simulink model "set_speed"  (R2021b)
settings: Solver=FixedStepDiscrete  StartTime=0.0  StopTime=inf  FixedStep=0.05  RelTol=1e-3
InitFcn:
  | ONE_FLOAT=1;
  | KVDI_ACCSetSpdIntial_kph=30;
  | KVDI_ACCLongPressTime_ms=3000;
  | KVDI_LongPressConTime_ms=800;
  | KVDI_ACCSpdLargeChange_kph=5;
  | ZERO_FLOAT=0;
  | FALSE=0;
  | TRUE=1;
  | ENUM_ACCSTATE_OFF=0;
  | ENUM_ACCSTATE_DISABLED=0;
  | ENUM_ACCSTATE_STANDBY=1;
  | KVDI_ACCMaxActSpeed_kph=150;
  | ONE_INT=1;
  | ZERO_INT=0;
  | C_TICK_TIME_S=0.05;
libraries: realtime_pacer_lib x1, simulink x1
settings Model: Creator=ZHEN-YU  LastModifiedBy=ZHEN-YU

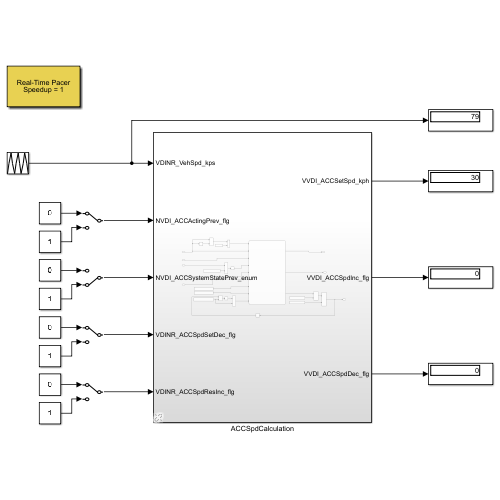
[thumbnail: Simulink's stored preview of the top-level diagram]
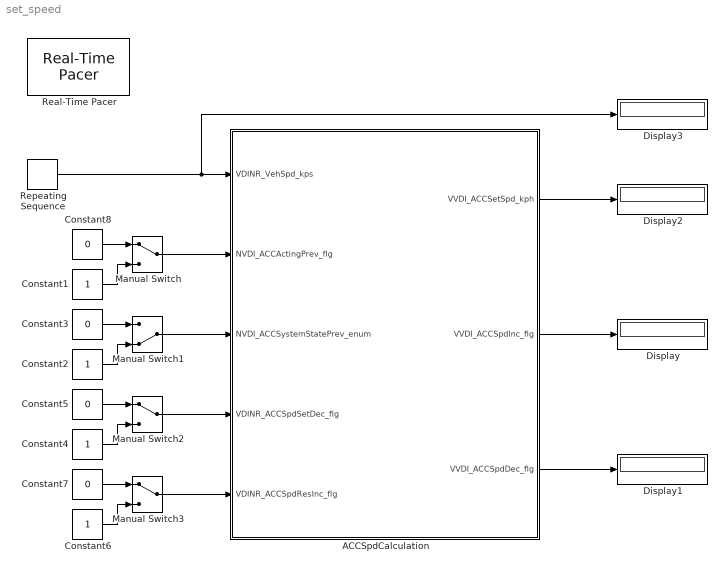
== system set_speed ==
  ACCSpdCalculation : Subsystem  AncestorBlock=vdi_v5/IFO/VDI/ACC/ACCSpdCalculation
  Constant{1..2,4,6} (4 alike) : Constant  OutDataTypeStr=boolean
  Constant{3,5,7..8} (4 alike) : Constant  Value=0  OutDataTypeStr=boolean
  Display{,1..3} (4 alike) : Display
  Manual Switch : ManualSwitch
  Manual Switch1 : ManualSwitch  CurrentSetting=0
  Manual Switch2 : ManualSwitch
  Manual Switch3 : ManualSwitch
  Real-Time Pacer : realtime_pacer_lib/Real-Time Pacer  simTimePerRealTime=1
  Repeating Sequence : simulink/Sources/Repeating Sequence  rep_seq_t=[0 10 20 30 40]  rep_seq_y=[0 50 100 50 0]
  wires:
  Repeating Sequence/1 -> Display3/1, ACCSpdCalculation/1(VDINR_VehSpd_kps)
  ACCSpdCalculation/2(VVDI_ACCSpdInc_flg) -> Display/1
  ACCSpdCalculation/3(VVDI_ACCSpdDec_flg) -> Display1/1
  ACCSpdCalculation/1(VVDI_ACCSetSpd_kph) -> Display2/1
  Constant8/1 -> Manual Switch/1
  Constant1/1 -> Manual Switch/2
  Manual Switch/1 -> ACCSpdCalculation/2(NVDI_ACCActingPrev_flg)
  Constant2/1 -> Manual Switch1/2
  Constant3/1 -> Manual Switch1/1
  Manual Switch1/1 -> ACCSpdCalculation/3(NVDI_ACCSystemStatePrev_enum)
  Constant5/1 -> Manual Switch2/1
  Constant4/1 -> Manual Switch2/2
  Manual Switch2/1 -> ACCSpdCalculation/4(VDINR_ACCSpdSetDec_flg)
  Manual Switch3/1 -> ACCSpdCalculation/5(VDINR_ACCSpdResInc_flg)
  Constant6/1 -> Manual Switch3/2
  Constant7/1 -> Manual Switch3/1

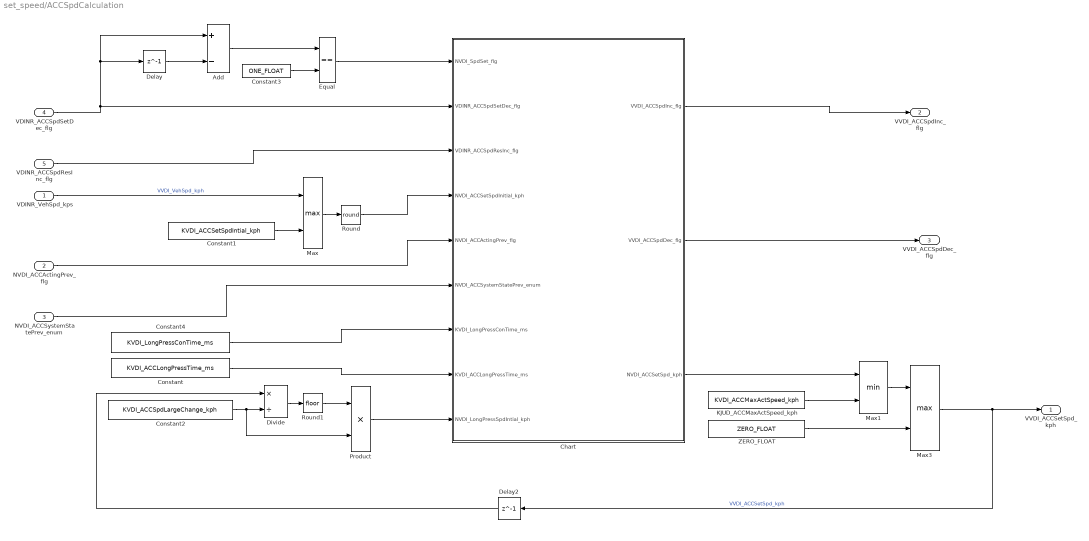
== system set_speed/ACCSpdCalculation ==
  VDINR_VehSpd_kps : Inport
  NVDI_ACCActingPrev_flg : Inport  Port=2
  NVDI_ACCSystemStatePrev_enum : Inport  Port=3
  VDINR_ACCSpdSetDec_flg : Inport  Port=4
  VDINR_ACCSpdResInc_flg : Inport  Port=5
  Add : Sum  Inputs=+-
  Chart : Stateflow chart  TreatAsAtomicUnit=on
      settings: PortSchema="{\"entries\":[{\"content\":{\"sides\":[{\"content\":{\"connectorIds\":[\"In1\",\"In2\",\"In3\",\"In4\",\"In5\",\"In6\",\"In9\",\"In7\",\"In8\"]},\"type\":\"ConnectorPlacement.EquallySpacedRectSide\",\"uuid\":\"b1b09059-7c6b-4f2a-a509-9d89abb69bff\"},{\"content\":{\"connectorIds\":[\"Out2\",\"Out3\",\"Out1\"],\"side\":\"RIGHT\"},\"type\":\"ConnectorPlacement.EquallySpacedRectSide\",\"uuid\":\"426eb2b7-8f84-437e-9ce1-b8172d5a5373\"},{\"content\":{\"connectorIds\":[],\"side\":\"TOP\"},\"type\":\"ConnectorPlacement.EquallySpacedRectSide\",\"uuid\":\"808310a0-6f78-4728-b2e8-69880cb1a9d0\"}]},\"type\":\"ConnectorPlacement.EquallySpacedConnector\",\"uuid\":\"50fcbb31-1c9a-4815-926e-b0772552613f\"}],\"packageUris\":[\"http://schema.mathworks.com/mf0/Connector/R2020b\"],\"version\":\"1.0\"}"
  Constant : Constant  Value=KVDI_ACCLongPressTime_ms
  Constant1 : Constant  Value=KVDI_ACCSetSpdIntial_kph
  Constant2 : Constant  Value=KVDI_ACCSpdLargeChange_kph
  Constant3 : Constant  Value=ONE_FLOAT
  Constant4 : Constant  Value=KVDI_LongPressConTime_ms
  Delay : Delay  DelayLength=1
  Delay2 : Delay  DelayLength=1
  Divide : Product  Inputs=*/
  Equal : RelationalOperator  Operator===  OutDataTypeStr=boolean  RndMeth=Simplest
  KJUD_ACCMaxActSpeed_kph : Constant  Value=KVDI_ACCMaxActSpeed_kph
  Max : MinMax  Function=max  Inputs=2
  Max1 : MinMax  Inputs=2
  Max3 : MinMax  Function=max  Inputs=2
  Product : Product
  Round : Rounding  Operator=round
  Round1 : Rounding
  ZERO_FLOAT : Constant  Value=ZERO_FLOAT
  VVDI_ACCSetSpd_kph : Outport
  VVDI_ACCSpdInc_flg : Outport  Port=2
  VVDI_ACCSpdDec_flg : Outport  Port=3
  wires:
  Constant/1 -> Chart/7(KVDI_ACCLongPressTime_ms)
  VDINR_ACCSpdResInc_flg/1 -> Chart/3(VDINR_ACCSpdResInc_flg)
  Max3/1 -> Delay2/1, VVDI_ACCSetSpd_kph/1  "VVDI_ACCSetSpd_kph"
  NVDI_ACCActingPrev_flg/1 -> Chart/5(NVDI_ACCActingPrev_flg)
  NVDI_ACCSystemStatePrev_enum/1 -> Chart/6(NVDI_ACCSystemStatePrev_enum)
  Max/1 -> Round/1
  Constant1/1 -> Max/2
  VDINR_VehSpd_kps/1 -> Max/1  "VVDI_VehSpd_kph"
  Round/1 -> Chart/4(NVDI_ACCSetSpdInitial_kph)
  Delay2/1 -> Divide/1
  Constant2/1 -> Product/2, Divide/2
  Round1/1 -> Product/1
  Divide/1 -> Round1/1
  Product/1 -> Chart/8(NVDI_LongPressSpdIntial_kph)
  Chart/1(NVDI_ACCSetSpd_kph) -> Max1/1
  ZERO_FLOAT/1 -> Max3/2
  Equal/1 -> Chart/1(NVDI_SpdSet_flg)
  Add/1 -> Equal/1
  Delay/1 -> Add/2
  Constant3/1 -> Equal/2
  VDINR_ACCSpdSetDec_flg/1 -> Add/1, Delay/1, Chart/2(VDINR_ACCSpdSetDec_flg)
  KJUD_ACCMaxActSpeed_kph/1 -> Max1/2
  Max1/1 -> Max3/1
  Chart/3(VVDI_ACCSpdDec_flg) -> VVDI_ACCSpdDec_flg/1
  Chart/2(VVDI_ACCSpdInc_flg) -> VVDI_ACCSpdInc_flg/1
  Constant4/1 -> Chart/9(KVDI_LongPressConTime_ms)

== stateflow chart set_speed/ACCSpdCalculation/Chart ==
  state INITIALIZATION
    en:
    NVDI_ACCSetSpd_kph = ZERO_INT;
    NVDI_ACCResSpd_kph=ZERO_INT;
    VVDI_ACCSpdDec_flg=FALSE;
    VVDI_ACCSpdInc_flg=FALSE;
  state STANDBY
    en:
    VVDI_ACCSpdDec_flg=FALSE;
    VVDI_ACCSpdInc_flg=FALSE;
    state Initial
      du:
      NVDI_ACCSetSpd_kph=NVDI_ACCSetSpdInitial_kph
    state Resume
      en:
      NVDI_ACCSetSpd_kph=NVDI_ACCResSpd_kph
    state Setting
      en:
      NVDI_ACCSetSpd_kph=NVDI_ACCSetSpdInitial_kph
    (default) -> Initial
    Initial -> Resume [order 2] : [VDINR_ACCSpdResInc_flg==TRUE...
        | &&NVDI_ACCResSpd_kph~=ZERO_INT]
    Resume -> Setting : [NVDI_SpdSet_flg==TRUE]
    Setting -> Resume : [VDINR_ACCSpdResInc_flg==TRUE...
        | &&NVDI_ACCResSpd_kph~=ZERO_INT]
    Initial -> Setting [order 1] : [NVDI_SpdSet_flg==TRUE]
  state SPEED_MODIF
    state Inc_Speed
      du:
      NVDI_ACCResSpd_kph=NVDI_ACCSetSpd_kph;
      VVDI_ACCSpdInc_flg=TRUE;
      state Small_Inc
        en:
        NVDI_ACCSetSpd_kph=NVDI_ACCSetSpd_kph+ONE_INT;
        NVDI_ACCIncTimer_ms=ZERO_INT;
        du:
        NVDI_ACCIncTimer_ms=NVDI_ACCIncTimer_ms+(C_TICK_TIME_S*1000);
      state Large_Inc_Frist
        en:
        NVDI_ACCSetSpd_kph=NVDI_LongPressSpdIntial_kph+KVDI_ACCSpdLargeChange_kph
      state MAINTAIN
        en:
        NVDI_ACCIncTimer_ms=ZERO_INT;
        du:
        NVDI_ACCIncTimer_ms=NVDI_ACCIncTimer_ms+(C_TICK_TIME_S*1000);
      state Large_Inc
        en:
        NVDI_ACCSetSpd_kph=NVDI_ACCSetSpd_kph+KVDI_ACCSpdLargeChange_kph
      (default) -> Small_Inc
      Small_Inc -> Large_Inc_Frist : [NVDI_ACCIncTimer_ms>KVDI_ACCLongPressTime_ms]
      Large_Inc_Frist -> SPEED_MODIF.Inc_Speed.MAINTAIN
      SPEED_MODIF.Inc_Speed.MAINTAIN -> Large_Inc : [NVDI_ACCIncTimer_ms>KVDI_LongPressConTime_ms]
      Large_Inc -> SPEED_MODIF.Inc_Speed.MAINTAIN
    state Dec_Speed
      du:
      NVDI_ACCResSpd_kph=NVDI_ACCSetSpd_kph;
      VVDI_ACCSpdDec_flg=TRUE;
      state Small_Dec
        en:
        NVDI_ACCSetSpd_kph=NVDI_ACCSetSpd_kph-ONE_INT;
        NVDI_ACCDecTimer_ms=ZERO_INT;
        du:
        NVDI_ACCDecTimer_ms=NVDI_ACCDecTimer_ms+(C_TICK_TIME_S*1000);
      state Large_Dec_Frist
        en:
        NVDI_ACCSetSpd_kph=NVDI_LongPressSpdIntial_kph
      state MAINTAIN
        en:
        NVDI_ACCDecTimer_ms=ZERO_INT;
        du:
        NVDI_ACCDecTimer_ms=NVDI_ACCDecTimer_ms+(C_TICK_TIME_S*1000);
      state Large_Dec
        en:
        NVDI_ACCSetSpd_kph=NVDI_ACCSetSpd_kph-KVDI_ACCSpdLargeChange_kph
      (default) -> Small_Dec
      Small_Dec -> Large_Dec_Frist : [NVDI_ACCDecTimer_ms>KVDI_ACCLongPressTime_ms]
      Large_Dec_Frist -> SPEED_MODIF.Dec_Speed.MAINTAIN
      Large_Dec -> SPEED_MODIF.Dec_Speed.MAINTAIN
      SPEED_MODIF.Dec_Speed.MAINTAIN -> Large_Dec : [NVDI_ACCDecTimer_ms>KVDI_LongPressConTime_ms]
    state HOLD
      en:
      NVDI_ACCSetSpd_kph=NVDI_ACCSetSpd_kph
      NVDI_ACCResSpd_kph=NVDI_ACCSetSpd_kph;
      VVDI_ACCSpdDec_flg=FALSE;
      VVDI_ACCSpdInc_flg=FALSE;
    (default) -> HOLD
    HOLD -> Dec_Speed [order 1] : [VDINR_ACCSpdSetDec_flg==TRUE]
    HOLD -> Inc_Speed [order 2] : [VDINR_ACCSpdResInc_flg==TRUE]
    Dec_Speed -> HOLD : [VDINR_ACCSpdSetDec_flg==FALSE]
    Inc_Speed -> HOLD : [VDINR_ACCSpdResInc_flg==FALSE]
  (default) -> INITIALIZATION
  INITIALIZATION -> STANDBY : [NVDI_ACCSystemStatePrev_enum == ENUM_ACCSTATE_STANDBY]
  STANDBY -> SPEED_MODIF [order 2] : [NVDI_ACCActingPrev_flg==TRUE]
  STANDBY -> INITIALIZATION [order 1] : [NVDI_ACCSystemStatePrev_enum == ENUM_ACCSTATE_OFF...
      | || NVDI_ACCSystemStatePrev_enum == ENUM_ACCSTATE_DISABLED]
  SPEED_MODIF -> STANDBY [order 2] : [NVDI_ACCActingPrev_flg==FALSE]
  SPEED_MODIF -> INITIALIZATION [order 1] : [NVDI_ACCSystemStatePrev_enum == ENUM_ACCSTATE_OFF...
      | || NVDI_ACCSystemStatePrev_enum == ENUM_ACCSTATE_DISABLED]
  data: NVDI_SpdSet_flg input; VDINR_ACCSpdSetDec_flg input; VDINR_ACCSpdResInc_flg input; NVDI_ACCSetSpdInitial_kph input; NVDI_ACCActingPrev_flg input; NVDI_ACCSystemStatePrev_enum input; NVDI_ACCSetSpd_kph output; KVDI_ACCLongPressTime_ms input; NVDI_LongPressSpdIntial_kph input; TRUE parameter boolean; ZERO_INT parameter; ONE_INT parameter; FALSE parameter boolean; ENUM_ACCSTATE_STANDBY parameter; ENUM_ACCSTATE_OFF parameter; ENUM_ACCSTATE_DISABLED parameter; C_TICK_TIME_S parameter; NVDI_ACCIncTimer_ms local; NVDI_ACCDecTimer_ms local; KVDI_ACCSpdLargeChange_kph parameter; NVDI_ACCResSpd_kph local; VVDI_ACCSpdInc_flg output; VVDI_ACCSpdDec_flg output; KVDI_LongPressConTime_ms input
